simulink model "PID_nonlinear_dynamics"  (R2022b)
settings: Solver=VariableStepAuto  StartTime=0.0  StopTime=20  RelTol=1e-3
values from neighbouring files (symbols this model uses):
  g = 9.8    [config.m]
  Jx = 2*Mc*R^2/5 + 2*m*l^2    (= 0.0448)    [config.m]
  Jy = 2*Mc*R^2/5 + 2*m*l^2    (= 0.0448)    [config.m]
  Jz = 2*Mc*R^2/5 + 4*m*l^2    (= 0.0808)    [config.m]
  Kd_pitch = 15    [config.m]
  Kd_roll = 15    [config.m]
  Kd_yaw = 15    [config.m]
  Kd_z = 15    [config.m]
  Ki_pitch = 1    [config.m]
  Ki_roll = 1    [config.m]
  Ki_yaw = 1    [config.m]
  Ki_z = 10    [config.m]
  Kp_pitch = 80    [config.m]
  Kp_roll = 80    [config.m]
  Kp_yaw = 80    [config.m]
  Kp_z = 80    [config.m]
  M = Mc + 4*m    (= 3)    [config.m]
libraries: simulink x2
settings Model: Creator=cxk  LastModifiedBy=cxk

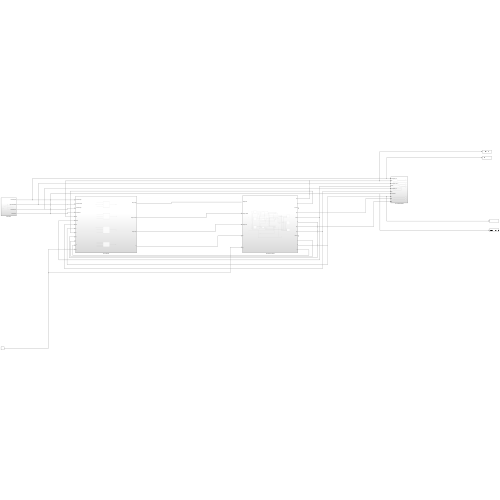
[thumbnail: Simulink's stored preview of the top-level diagram]
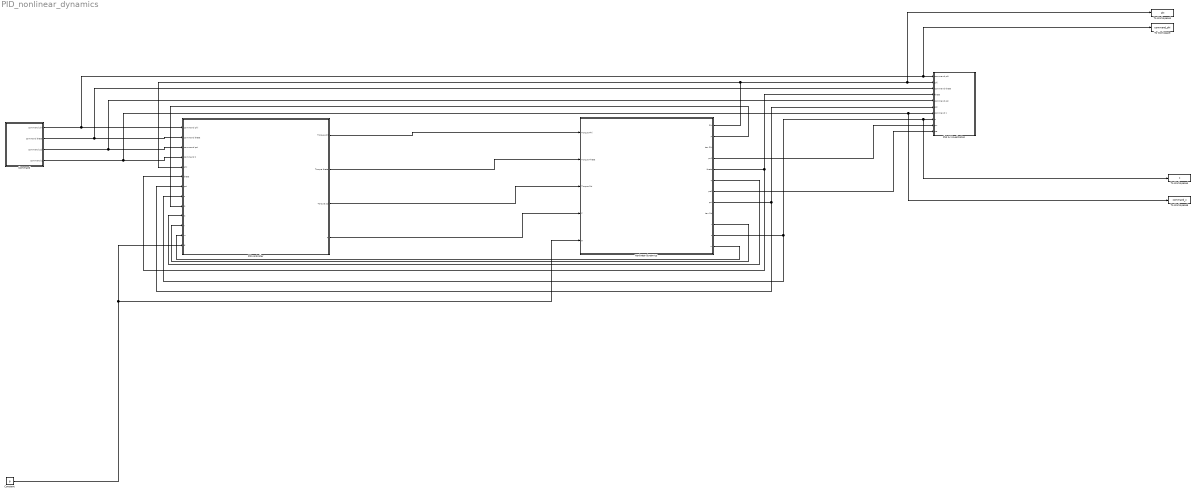
== system PID_nonlinear_dynamics ==
  Command : Subsystem
  Constant : Constant  Value=g
  Nonlinear dynamics : Subsystem
  PID controller : Subsystem
  Plot & Visualization : Subsystem
  To Workspace : ToWorkspace  VariableName=command_phi  SaveFormat=Timeseries  SampleTime=-1
  To Workspace1 : ToWorkspace  VariableName=phi  SaveFormat=Timeseries  SampleTime=-1
  To Workspace4 : ToWorkspace  VariableName=z  SaveFormat=Timeseries  SampleTime=-1
  To Workspace5 : ToWorkspace  VariableName=command_z  SaveFormat=Timeseries  SampleTime=-1
  wires:
  Constant/1 -> PID controller/13(g), Nonlinear dynamics/5(g)
  Nonlinear dynamics/8(psi) -> Plot & Visualization/6(psi), PID controller/7(psi)
  Nonlinear dynamics/5(theta) -> Plot & Visualization/4(theta), PID controller/6(theta)
  PID controller/4(F) -> Nonlinear dynamics/4(F)
  Nonlinear dynamics/2(p) -> PID controller/9(p)
  Nonlinear dynamics/6(q) -> PID controller/10(q)
  Nonlinear dynamics/10(r) -> PID controller/11(r)
  Nonlinear dynamics/12(w) -> PID controller/12(w)
  PID controller/1(Torque phi) -> Nonlinear dynamics/1(Torque Phi)
  PID controller/2(Torque theta) -> Nonlinear dynamics/2(Torque Theta)
  PID controller/3(Torque psi) -> Nonlinear dynamics/3(Torque Psi)
  Command/3(command psi) -> PID controller/3("command psi "), Plot & Visualization/5(command psi)
  Command/2(command theta) -> PID controller/2(command theta), Plot & Visualization/3(command theta)
  Nonlinear dynamics/4(pn1) -> Plot & Visualization/9(pn)
  Nonlinear dynamics/7(pe1) -> Plot & Visualization/10(pe)
  Nonlinear dynamics/11(z) -> PID controller/8(z), To Workspace4/1, Plot & Visualization/8(z)
  Command/4(command z) -> Plot & Visualization/7(command z), To Workspace5/1, PID controller/4(command z)
  Nonlinear dynamics/1(Phi) -> To Workspace1/1, Plot & Visualization/2(phi), PID controller/5(phi)
  Command/1(command phi) -> PID controller/1(command phi), To Workspace/1, Plot & Visualization/1(command phi)

== system PID_nonlinear_dynamics/Command ==
  Repeating Sequence1 : simulink/Sources/Repeating Sequence  rep_seq_t="[0 1 1.01  3 3.01 4 4.01 6]"  rep_seq_y=[0 0 1 1 -1 -1 0 0 ]
  Repeating Sequence2 : simulink/Sources/Repeating Sequence  rep_seq_t="[0 2 2.01  4 4.01 5 5.01 6]"  rep_seq_y=[0 0 1 1 -1 -1 0 0 ]
  Saturation4 : Saturate  UpperLimit=5  LowerLimit=-5
  Step : Step  After=0  SampleTime=0
  Step1 : Step  After=3  SampleTime=0
  pitch command : Sin  Amplitude=0  Frequency=0.5  SampleTime=0
  roll command : Sin  Amplitude=0  Frequency=0.5  SampleTime=0
  yaw command : Sin  Amplitude=pi  Frequency=0.5  SampleTime=0
  command phi : Outport
  command theta : Outport  Port=2
  command psi : Outport  Port=3
  command z : Outport  Port=4
  wires:
  Step1/1 -> Saturation4/1
  Saturation4/1 -> command z/1
  Step/1 -> command psi/1
  Repeating Sequence2/1 -> command phi/1
  Repeating Sequence1/1 -> command theta/1

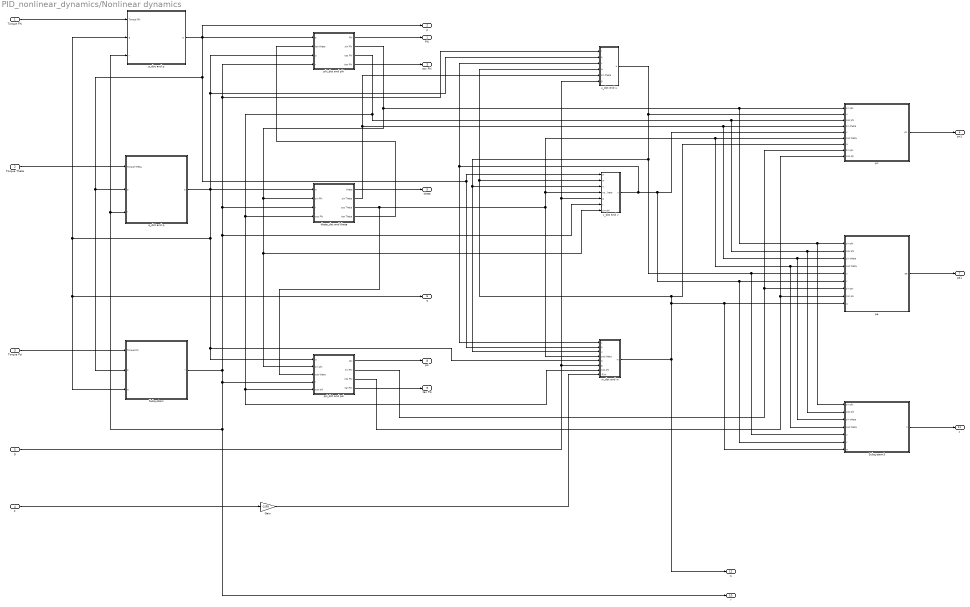
== system PID_nonlinear_dynamics/Nonlinear dynamics ==
  Torque Phi : Inport
  Torque Theta : Inport  Port=2
  Torque Psi : Inport  Port=3
  F : Inport  Port=4
  g : Inport  Port=5
  Gain : Gain  Gain=-1/M
  Subsystem : Subsystem
  Subsystem3 : Subsystem
  p_dot and p : Subsystem
  pe : Subsystem
  phi_dot and phi : Subsystem
  pn : Subsystem
  psi_dot and psi : Subsystem
  q_dot and q : Subsystem
  theta_dot and theta : Subsystem
  u_dot and u : Subsystem
  v_dot and v : Subsystem
  w_dot and w : Subsystem
  Phi : Outport
  p : Outport  Port=2
  tan Phi : Outport  Port=3
  pn1 : Outport  Port=4
  theta : Outport  Port=5
  q : Outport  Port=6
  pe1 : Outport  Port=7
  psi : Outport  Port=8
  tan Psi : Outport  Port=9
  r : Outport  Port=10
  z : Outport  Port=11
  w : Outport  Port=12
  wires:
  psi_dot and psi/3(cos Psi) -> pn/9(cos psi), pe/8(cos psi)
  phi_dot and phi/3(cos Phi) -> Subsystem3/2(cos phi), pe/2(cos phi), pn/3(cos phi), w_dot and w/7(cos phi), psi_dot and psi/5(cos phi), theta_dot and theta/4(cos Phi)
  theta_dot and theta/3(cos Theta) -> psi_dot and psi/3(cos theta), pn/6(cos theta), Subsystem3/4(cos theta), pe/4(cos theta), v_dot and v/4(cos theta), w_dot and w/4(cos theta)
  u_dot and u/1(u) -> Subsystem3/5(u), pe/5(u), w_dot and w/3(u), v_dot and v/3(u), pn/2(u)
  w_dot and w/1(w) -> w/1, Subsystem3/7(w), pe/9(w), pn/7(w), v_dot and v/2(w), u_dot and u/4(w)
  g/1 -> w_dot and w/6(g), v_dot and v/5(g), u_dot and u/6(g)
  theta_dot and theta/2(sin Theta) -> u_dot and u/5(sin theta), pn/4(sin theta), Subsystem3/3(sin theta), pe/3(sin theta)
  q_dot and q/1(q) -> w_dot and w/5(q), psi_dot and psi/1(q), q/1, Subsystem/3(q), p_dot and p/2(q), u_dot and u/2(q), phi_dot and phi/3(q), theta_dot and theta/1(q)
  phi_dot and phi/2(sin Phi) -> v_dot and v/7(sin phi), psi_dot and psi/2(sin phi), theta_dot and theta/2(sin Phi), pn/1(sin phi), Subsystem3/1(sin phi), pe/1(sin phi)
  v_dot and v/1(v) -> pn/5(v), Subsystem3/6(v), pe/6(v), u_dot and u/3(v), w_dot and w/1(v)
  Torque Theta/1 -> q_dot and q/1(Torque Theta)
  psi_dot and psi/2(sin Psi) -> pn/8(sin psi), pe/7(sin psi)
  theta_dot and theta/4(tan Theta) -> phi_dot and phi/2(tan theta)
  p_dot and p/1(p) -> w_dot and w/2(p), v_dot and v/1(p), q_dot and q/2(p), Subsystem/2(p), p/1, phi_dot and phi/1(p)
  pn/1(pn) -> pn1/1
  theta_dot and theta/1(theta) -> theta/1
  Subsystem/1(r) -> v_dot and v/6(r), u_dot and u/1(r), phi_dot and phi/4(r), theta_dot and theta/3(r), p_dot and p/3(r), q_dot and q/3(r), r/1, psi_dot and psi/4(r)
  psi_dot and psi/1(psi) -> psi/1
  Torque Phi/1 -> p_dot and p/1(Torque Phi)
  Torque Psi/1 -> Subsystem/1(Torque Psi)
  phi_dot and phi/1(Phi) -> Phi/1
  psi_dot and psi/4(tan Psi) -> tan Psi/1
  phi_dot and phi/4(tan Phi) -> tan Phi/1
  pe/1(pe) -> pe1/1
  Subsystem3/1(z) -> z/1
  F/1 -> Gain/1
  Gain/1 -> w_dot and w/8(-F/m)

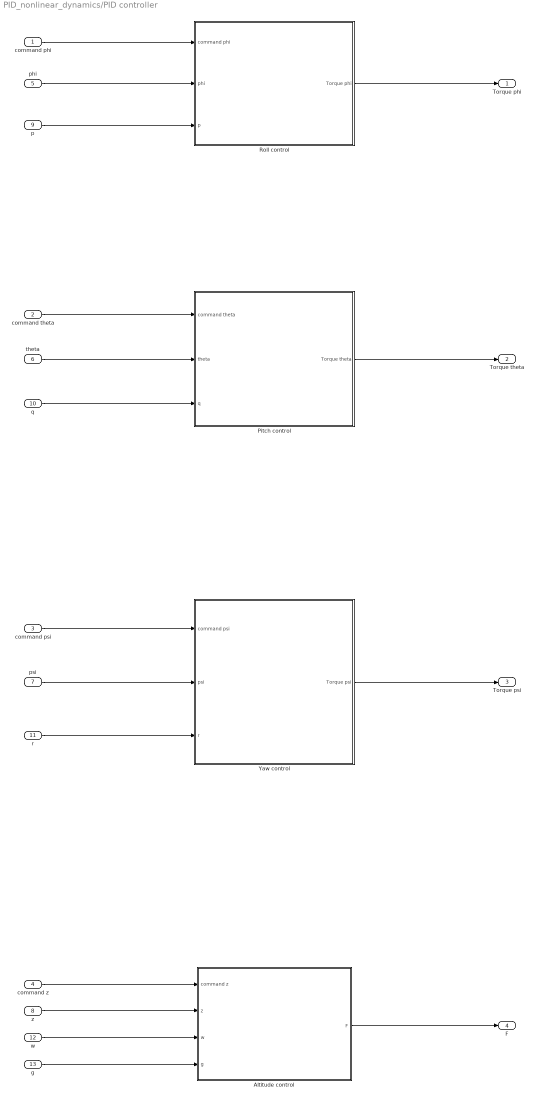
== system PID_nonlinear_dynamics/PID controller ==
  command phi : Inport
  command theta : Inport  Port=2
  "command psi " : Inport  Port=3
  command z : Inport  Port=4
  phi : Inport  Port=5
  theta : Inport  Port=6
  psi : Inport  Port=7
  z : Inport  Port=8
  p : Inport  Port=9
  q : Inport  Port=10
  r : Inport  Port=11
  w : Inport  Port=12
  g : Inport  Port=13
  Altitude control : Subsystem
  Pitch control : Subsystem
  Roll control : Subsystem
  Yaw control : Subsystem
  Torque phi : Outport
  Torque theta : Outport  Port=2
  Torque psi : Outport  Port=3
  F : Outport  Port=4
  wires:
  phi/1 -> Roll control/2(phi)
  command phi/1 -> Roll control/1(command phi)
  theta/1 -> Pitch control/2(theta)
  command theta/1 -> Pitch control/1(command theta)
  command z/1 -> Altitude control/1(command z)
  Yaw control/1(Torque psi) -> Torque psi/1
  z/1 -> Altitude control/2(z)
  "command psi "/1 -> Yaw control/1("command psi ")
  w/1 -> Altitude control/3(w)
  q/1 -> Pitch control/3(q)
  Altitude control/1(F) -> F/1
  Pitch control/1(Torque theta) -> Torque theta/1
  psi/1 -> Yaw control/2(psi)
  Roll control/1(Torque phi) -> Torque phi/1
  r/1 -> Yaw control/3(r)
  p/1 -> Roll control/3(p)
  g/1 -> Altitude control/4(g)

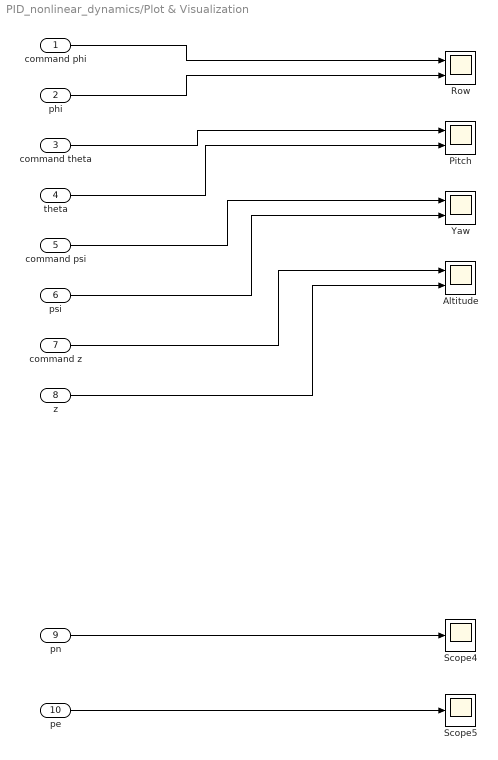
== system PID_nonlinear_dynamics/Plot & Visualization ==
  command phi : Inport
  phi : Inport  Port=2
  command theta : Inport  Port=3
  theta : Inport  Port=4
  command psi : Inport  Port=5
  psi : Inport  Port=6
  command z : Inport  Port=7
  z : Inport  Port=8
  pn : Inport  Port=9
  pe : Inport  Port=10
  Altitude : Scope  NumInputPorts=2
  Pitch : Scope  NumInputPorts=2
  Row : Scope  NumInputPorts=2
  Scope4 : Scope
  Scope5 : Scope
  Yaw : Scope  NumInputPorts=2
  wires:
  z/1 -> Altitude/2
  command phi/1 -> Row/1
  phi/1 -> Row/2
  command z/1 -> Altitude/1
  command psi/1 -> Yaw/1
  pe/1 -> Scope5/1
  psi/1 -> Yaw/2
  pn/1 -> Scope4/1
  theta/1 -> Pitch/2
  command theta/1 -> Pitch/1

== system PID_nonlinear_dynamics/Nonlinear dynamics/Subsystem ==
  note: $\dot r$
  note: ${(J_x-J_y) \over J_z}pq$
  note: r_dot and r
  note: $r$
  Torque Psi : Inport
  p : Inport  Port=2
  q : Inport  Port=3
  Gain2 : Gain  Gain=1/Jz
  Gain20 : Gain  Gain=(Jx-Jy)/Jz
  Integrator4 : Integrator
  Product2 : Product
  Sum11 : Sum
  r : Outport
  wires:
  Gain20/1 -> Product2/1
  Torque Psi/1 -> Gain2/1
  p/1 -> Gain20/1
  Sum11/1 -> Integrator4/1
  Product2/1 -> Sum11/2
  q/1 -> Product2/2
  Integrator4/1 -> r/1
  Gain2/1 -> Sum11/1

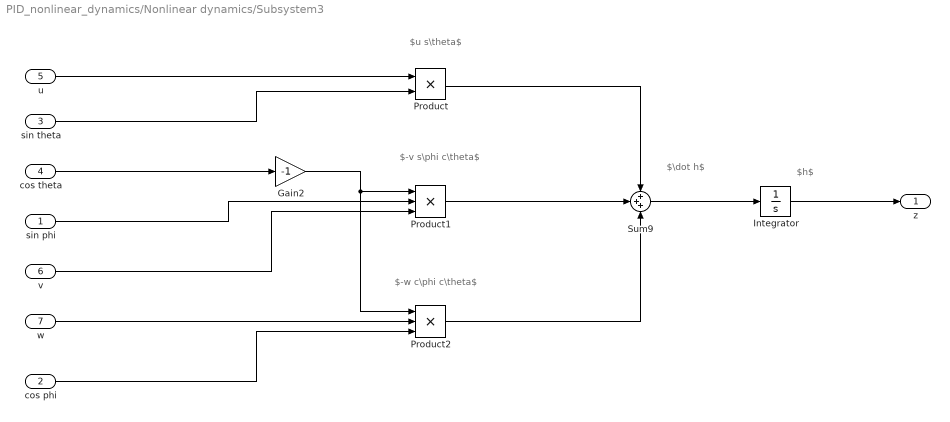
== system PID_nonlinear_dynamics/Nonlinear dynamics/Subsystem3 ==
  note: $u s\theta$
  note: $-v s\phi c\theta$
  note: $-w c\phi c\theta$
  note: $\dot h$
  note: $h$
  sin phi : Inport
  cos phi : Inport  Port=2
  sin theta : Inport  Port=3
  cos theta : Inport  Port=4
  u : Inport  Port=5
  v : Inport  Port=6
  w : Inport  Port=7
  Gain2 : Gain  Gain=-1
  Integrator : Integrator
  Product : Product
  Product1 : Product  Inputs=3
  Product2 : Product  Inputs=3
  Sum9 : Sum  Inputs=+++
  z : Outport
  wires:
  v/1 -> Product1/3
  Product1/1 -> Sum9/2
  Gain2/1 -> Product1/1, Product2/1
  cos phi/1 -> Product2/3
  u/1 -> Product/1
  sin phi/1 -> Product1/2
  Product/1 -> Sum9/1
  Product2/1 -> Sum9/3
  w/1 -> Product2/2
  sin theta/1 -> Product/2
  cos theta/1 -> Gain2/1
  Sum9/1 -> Integrator/1
  Integrator/1 -> z/1

== system PID_nonlinear_dynamics/Nonlinear dynamics/p_dot and p ==
  note: p_dot and p
  note: ${(J_y-J_z) \over J_x}qr$
  note: $\dot p$
  note: $p$
  Torque Phi : Inport
  q : Inport  Port=2
  r : Inport  Port=3
  Gain12 : Gain  Gain=1/Jx
  Gain17 : Gain  Gain=(Jy-Jz)/Jx
  Integrator2 : Integrator
  Product : Product
  Sum9 : Sum
  p : Outport
  wires:
  Sum9/1 -> Integrator2/1
  Product/1 -> Sum9/2
  r/1 -> Product/2
  Integrator2/1 -> p/1
  Gain17/1 -> Product/1
  Gain12/1 -> Sum9/1
  Torque Phi/1 -> Gain12/1
  q/1 -> Gain17/1

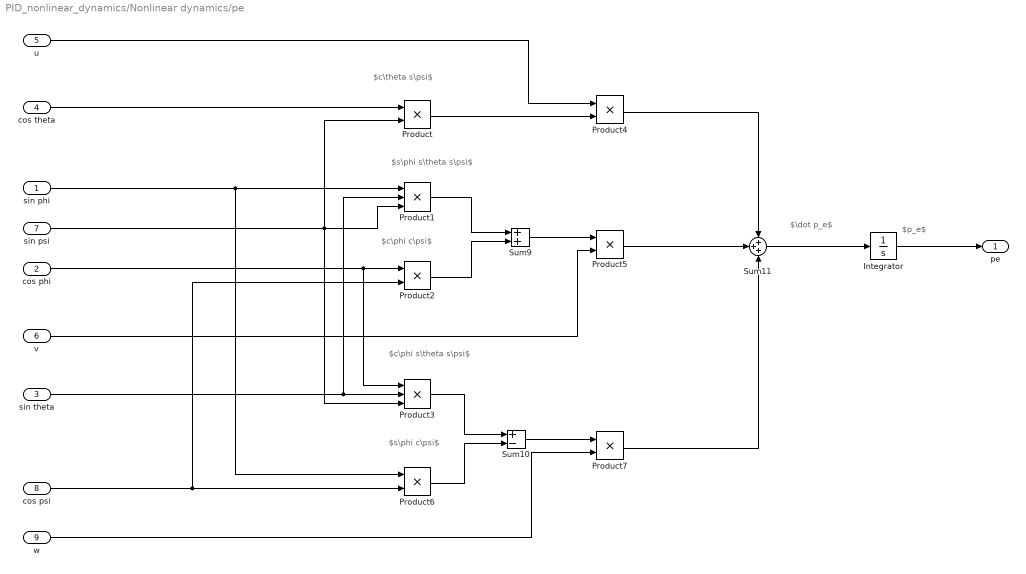
== system PID_nonlinear_dynamics/Nonlinear dynamics/pe ==
  note: $c\phi s\theta s\psi$
  note: $c\phi c\psi$
  note: $c\theta s\psi$
  note: $s\phi s\theta s\psi$
  note: $s\phi c\psi$
  note: $\dot p_e$
  note: $p_e$
  sin phi : Inport
  cos phi : Inport  Port=2
  sin theta : Inport  Port=3
  cos theta : Inport  Port=4
  u : Inport  Port=5
  v : Inport  Port=6
  sin psi : Inport  Port=7
  cos psi : Inport  Port=8
  w : Inport  Port=9
  Integrator : Integrator
  Product{,2,4..7} (6 alike) : Product
  Product1 : Product  Inputs=3
  Product3 : Product  Inputs=3
  Sum10 : Sum  Inputs=+-
  Sum11 : Sum  Inputs=+++
  Sum9 : Sum
  pe : Outport
  wires:
  sin psi/1 -> Product/2, Product1/3, Product3/3
  sin phi/1 -> Product1/1, Product6/1
  Sum9/1 -> Product5/1
  Product6/1 -> Sum10/2
  cos psi/1 -> Product6/2, Product2/2
  Product4/1 -> Sum11/1
  cos phi/1 -> Product3/1, Product2/1
  Product/1 -> Product4/2
  u/1 -> Product4/1
  Product5/1 -> Sum11/2
  w/1 -> Product7/2
  Sum11/1 -> Integrator/1
  sin theta/1 -> Product1/2, Product3/2
  Sum10/1 -> Product7/1
  Product7/1 -> Sum11/3
  Product1/1 -> Sum9/1
  Product2/1 -> Sum9/2
  Product3/1 -> Sum10/1
  cos theta/1 -> Product/1
  v/1 -> Product5/2
  Integrator/1 -> pe/1

== system PID_nonlinear_dynamics/Nonlinear dynamics/phi_dot and phi ==
  note: $\phi$
  note: $q*sin\phi*tan\theta$
  note: $r*cos\phi*tan\theta$
  note: $\dot \phi$
  p : Inport
  tan theta : Inport  Port=2
  q : Inport  Port=3
  r : Inport  Port=4
  Integrator1 : Integrator
  Product : Product  Inputs=3
  Product1 : Product  Inputs=3
  Subsystem1 : Subsystem
  Sum9 : Sum  Inputs=+++
  Phi : Outport
  sin Phi : Outport  Port=2
  cos Phi : Outport  Port=3
  tan Phi : Outport  Port=4
  wires:
  Subsystem1/2(cos Phi) -> cos Phi/1, Product1/2
  Subsystem1/1(sin Phi) -> sin Phi/1, Product/2
  q/1 -> Product/1
  Integrator1/1 -> Phi/1, Subsystem1/1(phi)
  Product/1 -> Sum9/2
  Sum9/1 -> Integrator1/1
  Product1/1 -> Sum9/3
  Subsystem1/3(tan Phi) -> tan Phi/1
  r/1 -> Product1/1
  p/1 -> Sum9/1
  tan theta/1 -> Product1/3, Product/3

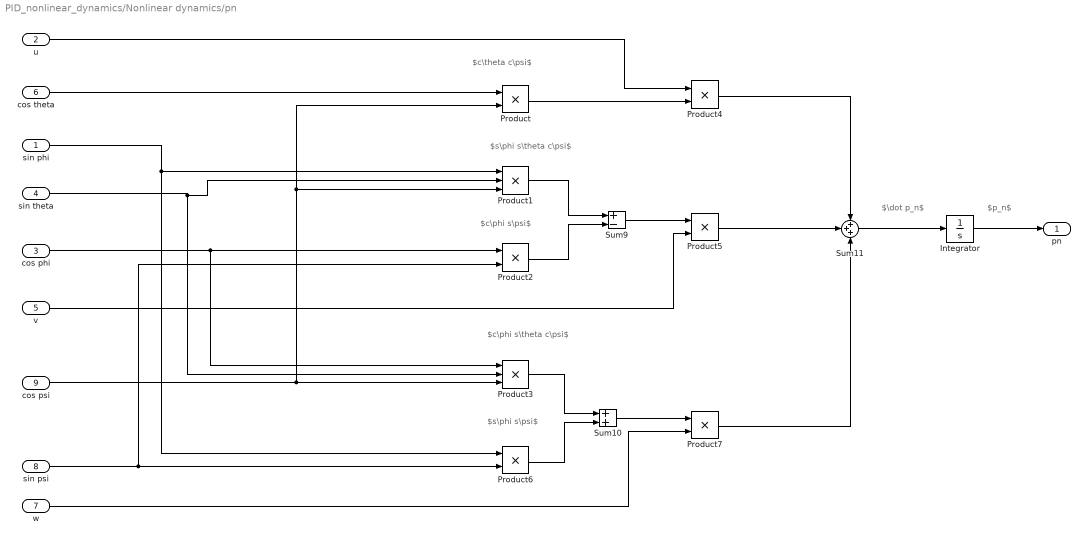
== system PID_nonlinear_dynamics/Nonlinear dynamics/pn ==
  note: $c\theta c\psi$
  note: $s\phi s\theta c\psi$
  note: $c\phi s\psi$
  note: $c\phi s\theta c\psi$
  note: $s\phi s\psi$
  note: $\dot p_n$
  note: $p_n$
  sin phi : Inport
  u : Inport  Port=2
  cos phi : Inport  Port=3
  sin theta : Inport  Port=4
  v : Inport  Port=5
  cos theta : Inport  Port=6
  w : Inport  Port=7
  sin psi : Inport  Port=8
  cos psi : Inport  Port=9
  Integrator : Integrator
  Product{,2,4..7} (6 alike) : Product
  Product1 : Product  Inputs=3
  Product3 : Product  Inputs=3
  Sum10 : Sum
  Sum11 : Sum  Inputs=+++
  Sum9 : Sum  Inputs=+-
  pn : Outport
  wires:
  cos phi/1 -> Product3/1, Product2/1
  Product4/1 -> Sum11/1
  Sum9/1 -> Product5/1
  Sum11/1 -> Integrator/1
  cos psi/1 -> Product3/3, Product1/3, Product/2
  sin theta/1 -> Product3/2, Product1/2
  sin psi/1 -> Product2/2, Product6/2
  Product5/1 -> Sum11/2
  Product3/1 -> Sum10/1
  Product2/1 -> Sum9/2
  Product6/1 -> Sum10/2
  sin phi/1 -> Product6/1, Product1/1
  Product1/1 -> Sum9/1
  Sum10/1 -> Product7/1
  Product/1 -> Product4/2
  Product7/1 -> Sum11/3
  u/1 -> Product4/1
  v/1 -> Product5/2
  cos theta/1 -> Product/1
  w/1 -> Product7/2
  Integrator/1 -> pn/1

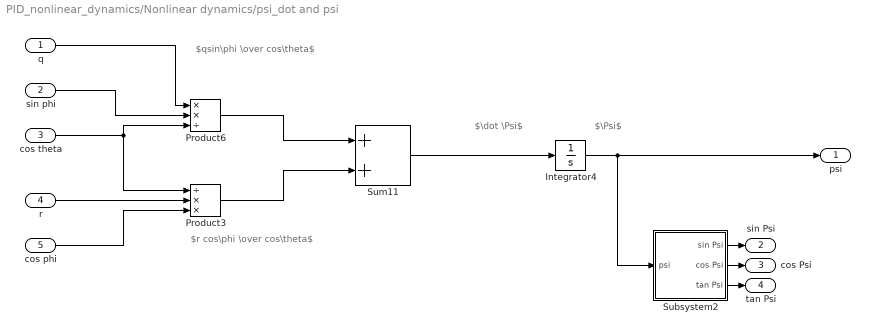
== system PID_nonlinear_dynamics/Nonlinear dynamics/psi_dot and psi ==
  note: $\Psi$
  note: $qsin\phi \over cos\theta$
  note: $r cos\phi \over cos\theta$
  note: $\dot \Psi$
  q : Inport
  sin phi : Inport  Port=2
  cos theta : Inport  Port=3
  r : Inport  Port=4
  cos phi : Inport  Port=5
  Integrator4 : Integrator
  Product3 : Product  Inputs=/**
  Product6 : Product  Inputs=**/
  Subsystem2 : Subsystem
  Sum11 : Sum  Inputs=+|+
  psi : Outport
  sin Psi : Outport  Port=2
  cos Psi : Outport  Port=3
  tan Psi : Outport  Port=4
  wires:
  Subsystem2/2(cos Psi) -> cos Psi/1
  Sum11/1 -> Integrator4/1
  Integrator4/1 -> psi/1, Subsystem2/1(psi)
  Product3/1 -> Sum11/2
  sin phi/1 -> Product6/2
  Product6/1 -> Sum11/1
  q/1 -> Product6/1
  cos theta/1 -> Product6/3, Product3/1
  Subsystem2/1(sin Psi) -> sin Psi/1
  Subsystem2/3(tan Psi) -> tan Psi/1
  r/1 -> Product3/2
  cos phi/1 -> Product3/3

== system PID_nonlinear_dynamics/Nonlinear dynamics/q_dot and q ==
  note: $\dot q$
  note: ${(J_z-J_x) \over J_y}pr$
  note: q_dot and q
  note: $q$
  Torque Theta : Inport
  p : Inport  Port=2
  r : Inport  Port=3
  Gain16 : Gain  Gain=1/Jy
  Gain19 : Gain  Gain=(Jz-Jx)/Jy
  Integrator1 : Integrator
  Product1 : Product
  Sum10 : Sum
  q : Outport
  wires:
  Gain16/1 -> Sum10/1
  Integrator1/1 -> q/1
  Sum10/1 -> Integrator1/1
  r/1 -> Product1/2
  Gain19/1 -> Product1/1
  Product1/1 -> Sum10/2
  Torque Theta/1 -> Gain16/1
  p/1 -> Gain19/1

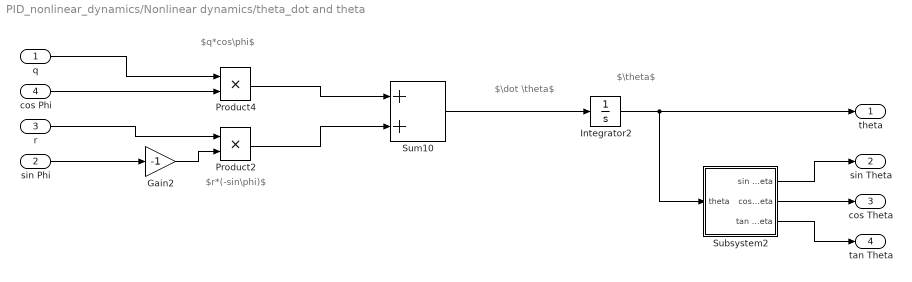
== system PID_nonlinear_dynamics/Nonlinear dynamics/theta_dot and theta ==
  note: $\theta$
  note: $q*cos\phi$
  note: $r*(-sin\phi)$
  note: $\dot \theta$
  q : Inport
  sin Phi : Inport  Port=2
  r : Inport  Port=3
  cos Phi : Inport  Port=4
  Gain2 : Gain  Gain=-1
  Integrator2 : Integrator
  Product2 : Product
  Product4 : Product
  Subsystem2 : Subsystem
  Sum10 : Sum  Inputs=+|+
  theta : Outport
  sin Theta : Outport  Port=2
  cos Theta : Outport  Port=3
  tan Theta : Outport  Port=4
  wires:
  r/1 -> Product2/1
  Subsystem2/1(sin Theta) -> sin Theta/1
  Product2/1 -> Sum10/2
  Sum10/1 -> Integrator2/1
  sin Phi/1 -> Gain2/1
  Gain2/1 -> Product2/2
  Integrator2/1 -> theta/1, Subsystem2/1(theta)
  Product4/1 -> Sum10/1
  cos Phi/1 -> Product4/2
  Subsystem2/3(tan Theta) -> tan Theta/1
  q/1 -> Product4/1
  Subsystem2/2(cos Theta) -> cos Theta/1

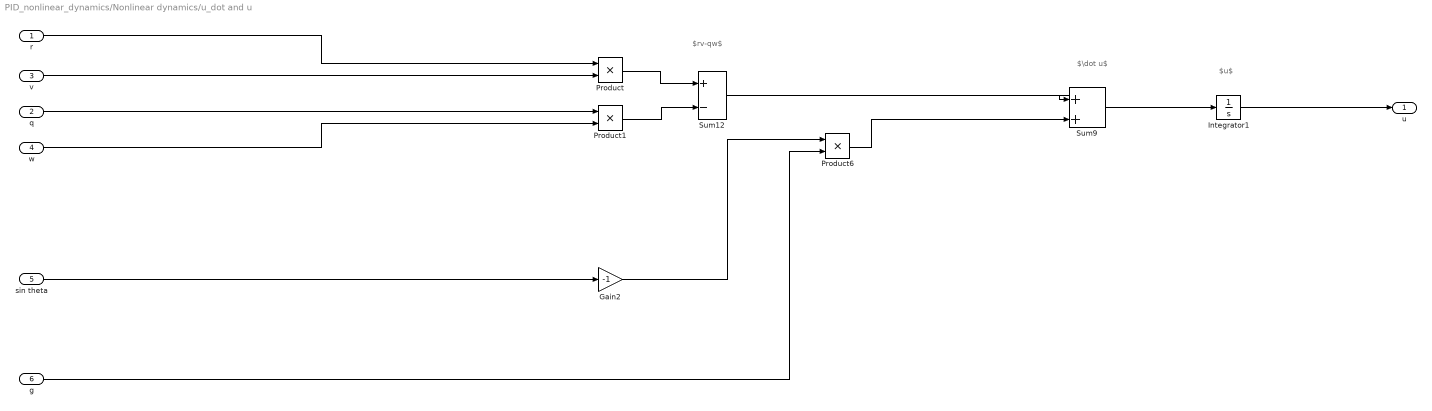
== system PID_nonlinear_dynamics/Nonlinear dynamics/u_dot and u ==
  note: $rv-qw$
  note: $\dot u$
  note: $u$
  r : Inport
  q : Inport  Port=2
  v : Inport  Port=3
  w : Inport  Port=4
  sin theta : Inport  Port=5
  g : Inport  Port=6
  Gain2 : Gain  Gain=-1
  Integrator1 : Integrator
  Product : Product
  Product1 : Product
  Product6 : Product
  Sum12 : Sum  Inputs=+|-
  Sum9 : Sum  Inputs=+|+
  u : Outport
  wires:
  Integrator1/1 -> u/1
  Sum9/1 -> Integrator1/1
  q/1 -> Product1/1
  Product1/1 -> Sum12/2
  Product/1 -> Sum12/1
  Product6/1 -> Sum9/2
  sin theta/1 -> Gain2/1
  Gain2/1 -> Product6/1
  Sum12/1 -> Sum9/1
  g/1 -> Product6/2
  v/1 -> Product/2
  r/1 -> Product/1
  w/1 -> Product1/2

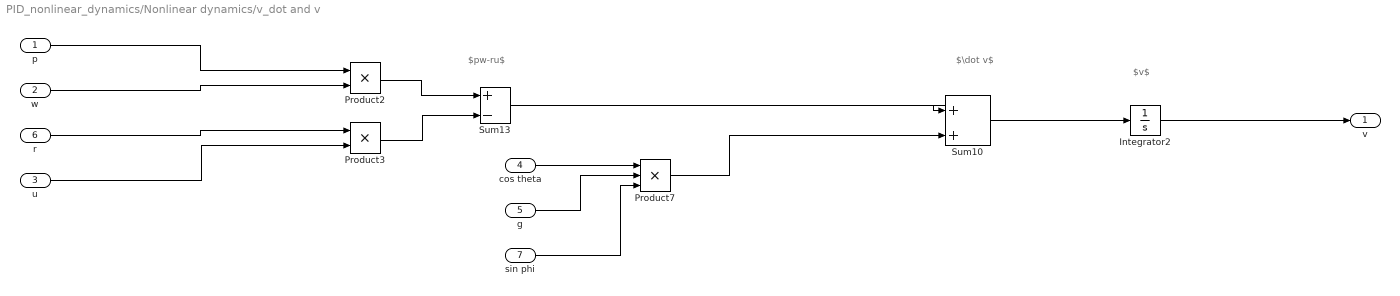
== system PID_nonlinear_dynamics/Nonlinear dynamics/v_dot and v ==
  note: $pw-ru$
  note: $\dot v$
  note: $v$
  p : Inport
  w : Inport  Port=2
  u : Inport  Port=3
  cos theta : Inport  Port=4
  g : Inport  Port=5
  r : Inport  Port=6
  sin phi : Inport  Port=7
  Integrator2 : Integrator
  Product2 : Product
  Product3 : Product
  Product7 : Product  Inputs=3
  Sum10 : Sum  Inputs=+|+
  Sum13 : Sum  Inputs=+|-
  v : Outport
  wires:
  cos theta/1 -> Product7/1
  Product3/1 -> Sum13/2
  Integrator2/1 -> v/1
  w/1 -> Product2/2
  Sum13/1 -> Sum10/1
  Sum10/1 -> Integrator2/1
  Product2/1 -> Sum13/1
  Product7/1 -> Sum10/2
  u/1 -> Product3/2
  g/1 -> Product7/2
  p/1 -> Product2/1
  sin phi/1 -> Product7/3
  r/1 -> Product3/1

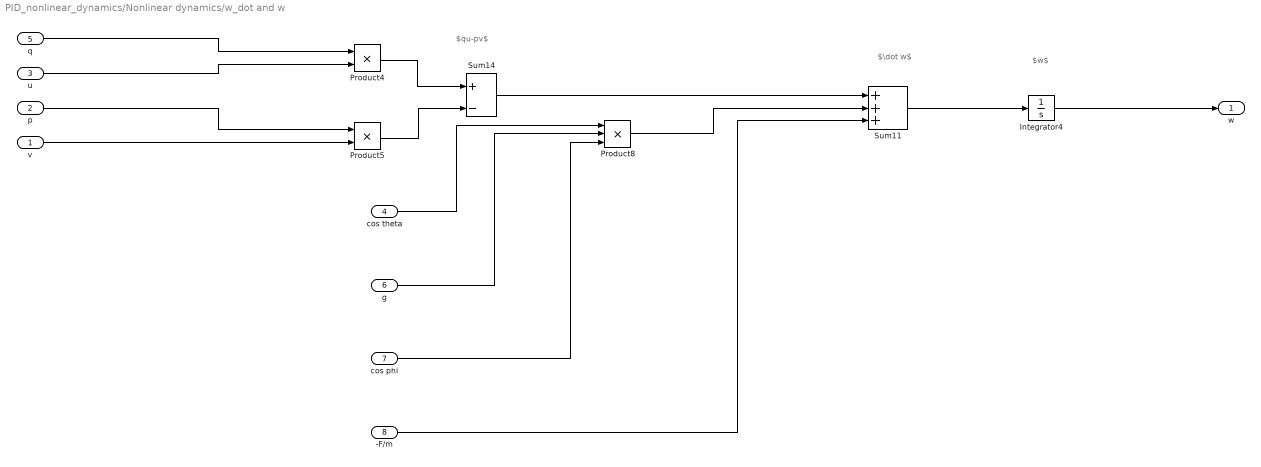
== system PID_nonlinear_dynamics/Nonlinear dynamics/w_dot and w ==
  note: $qu-pv$
  note: $\dot w$
  note: $w$
  v : Inport
  p : Inport  Port=2
  u : Inport  Port=3
  cos theta : Inport  Port=4
  q : Inport  Port=5
  g : Inport  Port=6
  cos phi : Inport  Port=7
  -F/m : Inport  Port=8
  Integrator4 : Integrator
  Product4 : Product
  Product5 : Product
  Product8 : Product  Inputs=3
  Sum11 : Sum  Inputs=+++
  Sum14 : Sum  Inputs=+|-
  w : Outport
  wires:
  cos phi/1 -> Product8/3
  Sum14/1 -> Sum11/1
  Product8/1 -> Sum11/2
  Product4/1 -> Sum14/1
  Sum11/1 -> Integrator4/1
  Product5/1 -> Sum14/2
  Integrator4/1 -> w/1
  -F/m/1 -> Sum11/3
  g/1 -> Product8/2
  p/1 -> Product5/1
  q/1 -> Product4/1
  v/1 -> Product5/2
  cos theta/1 -> Product8/1
  u/1 -> Product4/2

== system PID_nonlinear_dynamics/PID controller/Altitude control ==
  note: $F= {(g-\ddot{p_d})*M}$
  note: Error_z
  note: F
  command z : Inport
  z : Inport  Port=2
  w : Inport  Port=3
  g : Inport  Port=4
  Gain1 : Gain  Gain=M
  Gain10 : Gain  Gain=Ki_z
  Gain11 : Gain  Gain=Kd_z
  Gain9 : Gain  Gain=Kp_z
  Integrator9 : Integrator
  Saturation3 : Saturate  UpperLimit=g*M*10  LowerLimit=-2.97*M*10
  Sum6 : Sum  Inputs=|+-
  Sum7 : Sum  Inputs=|-+
  Sum8 : Sum  Inputs=++-
  F : Outport
  wires:
  Sum6/1 -> Gain1/1
  Sum7/1 -> Gain10/1, Gain9/1
  Gain9/1 -> Sum8/2
  Integrator9/1 -> Sum8/1
  g/1 -> Sum6/1
  Gain10/1 -> Integrator9/1
  Sum8/1 -> Sum6/2
  Gain1/1 -> Saturation3/1
  command z/1 -> Sum7/1
  Gain11/1 -> Sum8/3
  Saturation3/1 -> F/1
  z/1 -> Sum7/2
  w/1 -> Gain11/1

== system PID_nonlinear_dynamics/PID controller/Pitch control ==
  note: $E_\theta=\theta_d-\theta$
  note: $\tau_\theta$
  command theta : Inport
  theta : Inport  Port=2
  q : Inport  Port=3
  Gain13 : Gain  Gain=Kp_pitch
  Gain14 : Gain  Gain=Ki_pitch
  Gain15 : Gain  Gain=Kd_pitch
  Integrator3 : Integrator
  Saturation1 : Saturate  UpperLimit=100  LowerLimit=-100
  Sum2 : Sum  Inputs=|+-
  Sum3 : Sum  Inputs=++-
  Torque theta : Outport
  wires:
  command theta/1 -> Sum2/1
  Sum2/1 -> Gain14/1, Gain13/1
  Gain14/1 -> Integrator3/1
  Sum3/1 -> Saturation1/1
  Integrator3/1 -> Sum3/1
  Gain15/1 -> Sum3/3
  theta/1 -> Sum2/2
  Gain13/1 -> Sum3/2
  Saturation1/1 -> Torque theta/1
  q/1 -> Gain15/1

== system PID_nonlinear_dynamics/PID controller/Roll control ==
  note: $\tau_\phi$
  note: $E_\phi=\phi_d-\phi$
  command phi : Inport
  phi : Inport  Port=2
  p : Inport  Port=3
  Gain3 : Gain  Gain=Kp_roll
  Gain4 : Gain  Gain=Ki_roll
  Gain5 : Gain  Gain=Kd_roll
  Integrator : Integrator
  Saturation : Saturate  UpperLimit=100  LowerLimit=-100
  Sum : Sum  Inputs=|+-
  Sum1 : Sum  Inputs=++-
  Torque phi : Outport
  wires:
  Integrator/1 -> Sum1/1
  Sum/1 -> Gain4/1, Gain3/1
  Gain4/1 -> Integrator/1
  Gain5/1 -> Sum1/3
  Saturation/1 -> Torque phi/1
  Sum1/1 -> Saturation/1
  Gain3/1 -> Sum1/2
  command phi/1 -> Sum/1
  phi/1 -> Sum/2
  p/1 -> Gain5/1

== system PID_nonlinear_dynamics/PID controller/Yaw control ==
  note: $E_\Psi=\Psi-\Psi_d$
  note: $\tau_\psi$
  "command psi " : Inport
  psi : Inport  Port=2
  r : Inport  Port=3
  Gain6 : Gain  Gain=Kd_yaw
  Gain7 : Gain  Gain=Kp_yaw
  Gain8 : Gain  Gain=Ki_yaw
  Integrator7 : Integrator
  Saturation2 : Saturate  UpperLimit=100  LowerLimit=-100
  Sum4 : Sum  Inputs=---
  Sum5 : Sum  Inputs=|-+
  Torque psi : Outport
  wires:
  Sum4/1 -> Saturation2/1
  Integrator7/1 -> Sum4/1
  Gain8/1 -> Integrator7/1
  psi/1 -> Sum5/2
  Sum5/1 -> Gain8/1, Gain7/1
  Gain7/1 -> Sum4/2
  Gain6/1 -> Sum4/3
  "command psi "/1 -> Sum5/1
  Saturation2/1 -> Torque psi/1
  r/1 -> Gain6/1

== system PID_nonlinear_dynamics/Nonlinear dynamics/phi_dot and phi/Subsystem1 ==
  phi : Inport
  Trigonometric Function : Trigonometry
  Trigonometric Function1 : Trigonometry  Operator=cos
  Trigonometric Function2 : Trigonometry  Operator=tan
  sin Phi : Outport
  cos Phi : Outport  Port=2
  tan Phi : Outport  Port=3
  wires:
  phi/1 -> Trigonometric Function2/1, Trigonometric Function1/1, Trigonometric Function/1
  Trigonometric Function2/1 -> tan Phi/1
  Trigonometric Function/1 -> sin Phi/1
  Trigonometric Function1/1 -> cos Phi/1

== system PID_nonlinear_dynamics/Nonlinear dynamics/psi_dot and psi/Subsystem2 ==
  psi : Inport
  Trigonometric Function : Trigonometry
  Trigonometric Function1 : Trigonometry  Operator=cos
  Trigonometric Function2 : Trigonometry  Operator=tan
  sin Psi : Outport
  cos Psi : Outport  Port=2
  tan Psi : Outport  Port=3
  wires:
  psi/1 -> Trigonometric Function2/1, Trigonometric Function1/1, Trigonometric Function/1
  Trigonometric Function2/1 -> tan Psi/1
  Trigonometric Function/1 -> sin Psi/1
  Trigonometric Function1/1 -> cos Psi/1

== system PID_nonlinear_dynamics/Nonlinear dynamics/theta_dot and theta/Subsystem2 ==
  theta : Inport
  Trigonometric Function : Trigonometry
  Trigonometric Function1 : Trigonometry  Operator=cos
  Trigonometric Function2 : Trigonometry  Operator=tan
  sin Theta : Outport
  cos Theta : Outport  Port=2
  tan Theta : Outport  Port=3
  wires:
  theta/1 -> Trigonometric Function2/1, Trigonometric Function1/1, Trigonometric Function/1
  Trigonometric Function2/1 -> tan Theta/1
  Trigonometric Function/1 -> sin Theta/1
  Trigonometric Function1/1 -> cos Theta/1
